simulink model "MicroMouseTemplate"  (R2023a)
settings: Solver=FixedStepAuto  StartTime=0.0  StopTime=50  RelTol=1e-3  EnableMultiTasking=on
undefined symbols (not defined in the file or in its folder): samplingTime
settings Model: SimulationMode=external  ExtModeTrigDuration=10  Creator=JesseJabezArendse  LastModifiedBy=Dylan Howard
settings SolverCC: AllowMultiTaskInputOutput=on  AutoInsertRateTranBlk=on  InsertRTBMode=Never (minimum delay)
settings OptimizationCC: EnhancedBackFolding=on  PassReuseOutputArgsAs=Individual arguments  StateBitsets=on  DataBitsets=on  ZeroExternalMemoryAtStartup=off  ZeroInternalMemoryAtStartup=off  NoFixptDivByZeroProtection=on  MaxStackSize=64  OptimizeBlockOrder=speed  DifferentSizesBufferReuse=on  EfficientTunableParamExpr=on
settings DebuggingCC: MultiTaskCondExecSysMsg=none  ParameterOverflowMsg=none  ParameterPrecisionLossMsg=none  ParameterTunabilityLossMsg=error
settings HardwareCC: ProdBitPerPointer=32  ProdBitPerSizeT=32  ProdBitPerPtrDiffT=32  ProdLargestAtomicInteger=Long  ProdLargestAtomicFloat=Double  ProdWordSize=32  ProdLongLongMode=on  ProdHWDeviceType=ARM Compatible->ARM Cortex  TargetBitPerPointer=64  TargetBitPerSizeT=64  TargetBitPerPtrDiffT=64  TargetLongLongMode=on  TargetIntDivRoundTo=Zero  TargetEndianess=LittleEndian  TargetWordSize=64  TargetHWDeviceType=MATLAB Host
settings ModelReferenceCC: EnableParallelModelReferenceBuilds=on  ParallelModelReferenceMATLABWorkerInit=Copy Base Workspace  SupportModelReferenceSimTargetCustomCode=on
settings SFSimCC: MATLABDynamicMemAlloc=off  SimHardwareAcceleration=native
settings RTWCC: Description=Embedded Coder  SystemTargetFile=ert.tlc  HardwareBoard=STM32L4xx Based  TLCOptions=-p0 -aInlineSetEventsForThisBaseRateFcn=TLC_FALSE -aSuppressMultiTaskScheduler=TLC_FALSE -aRateBasedStepFcn=1  TemplateMakefile=ert_default_tmf  Toolchain=GNU Tools for ARM Embedded Processors  CodeExecutionProfiling=on  CodeProfilingInstrumentation=coarse
settings RTWCC: CustomHeaderCode=|
  | #include "MicroMouseProgramming\Core\Inc\IMU.h"
  | #include "MicroMouseProgramming\Core\Inc\CustomWhile.h"
  | #include "MicroMouseProgramming\Core\Inc\Motors.h"
settings RTWCC: CustomInclude=|
  | MicroMouseProgramming\Core\Inc\
  | MicroMouseProgramming\Core\Src\
settings RTWCC: CustomSource=|
  | MicroMouseProgramming\Core\Src\IMU.c
  | MicroMouseProgramming\Core\Src\CustomWhile.c
  | MicroMouseProgramming\Core\Src\Motors.c
settings CodeAppCC: ForceParamTrailComments=on  IgnoreCustomStorageClasses=off  OperatorAnnotations=on  SimulinkDataObjDesc=on  SFDataObjDesc=on  InsertBlockDesc=on
settings ERTTargetCC: CodeReplacementLibrary=ARM Cortex-M  SupportNonFinite=off  SupportComplex=off  ExtModeTransport=3  ExtModeStaticAlloc=on  ExtModeStaticAllocSize=2048  ExtModeMexFile=ext_xcp  ExtModeIntrfLevel=Level2 - Open

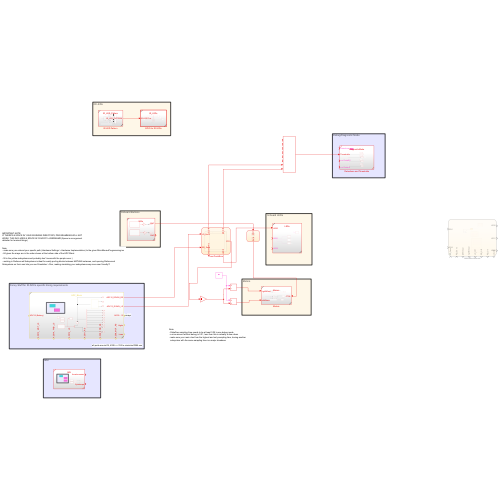
[thumbnail: Simulink's stored preview of the top-level diagram]
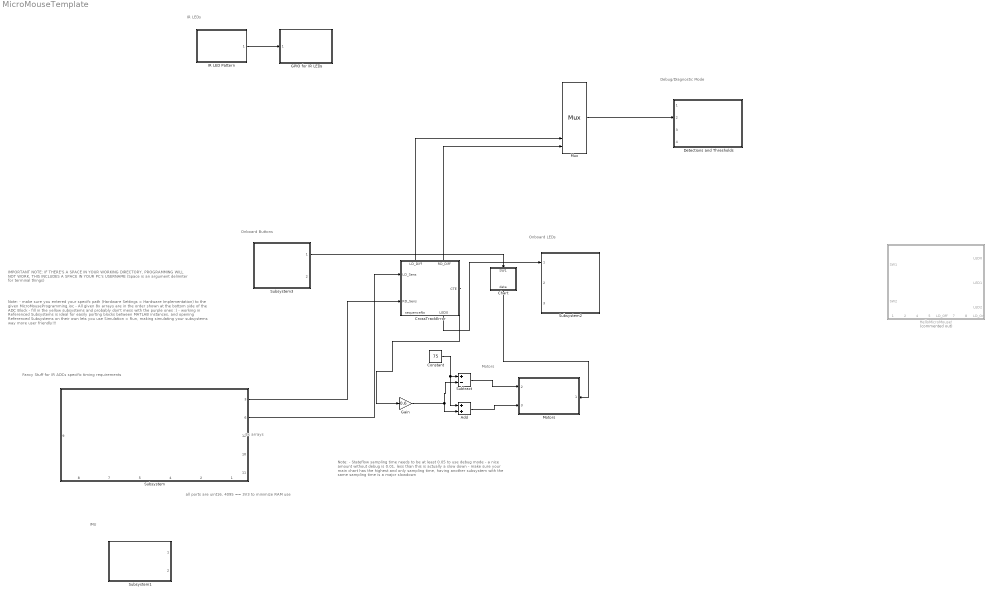
== system MicroMouseTemplate ==
  note: IMPORTANT NOTE:
      | IF THERE'S A SPACE IN YOUR WORKING DIRECTORY, PROGRAMMING WILL NOT WORK, THIS INCLUDES A SPACE IN YOUR PC's USERNAME (Space is an argument delimiter for terminal things)
  note: Note:
      | - make sure you entered your specifc path (Hardware Settings > Hardware Implementation) to the given MicroMouseProgramming.ioc
      | - All given 8x arrays are in the order shown at the bottom side of the ADC Block
      |
      | - fill in the yellow subsystems and probably don't mess with the purple ones :)
      | - working in Referenced Subsystems is ideal for easily porting blocks between MATLAB instances, and opening Referenced Subsystems on their own lets you use Simulation > Run, making simulating your subsystems way more user friendly!!!
  note: 8x arrays
  note: all ports are uint16, 4095 == 3V3 to minimize RAM use
  note: IMU
  note: Note:
      | - Stateflow sampling time needs to be at least 0.05 to use debug mode
      | - a nice amount without debug is 0.01, less than this is actually a slow down
      | - make sure your main chart has the highest and only sampling time, having another
      | subsystem with the same sampling time is a major slowdown
  note: Fancy Stuff for IR ADCs specific timing requirements
  note: IR LEDs
  note: Motors
  note: Onboard Buttons
  note: Onboard LEDs
  note: Debug/Diagnostic Mode
  Add : Sum
  Chart : Stateflow chart  TreatAsAtomicUnit=on
      settings: PortSchema="{\"entries\":[{\"content\":{\"sides\":[{\"content\":{},\"type\":\"ConnectorPlacement.EquallySpacedRectSide\",\"uuid\":\"65ce9c31-f788-4c01-8003-f22def2aa1a8\"},{\"content\":{\"side\":\"RIGHT\"},\"type\":\"ConnectorPlacement.EquallySpacedRectSide\",\"uuid\":\"9abbc0da-d05e-45e1-a3c7-84c2424ccecc\"},{\"content\":{\"connectorIds\":[\"In1\"],\"side\":\"TOP\"},\"type\":\"ConnectorPlacement.EquallySpacedRectSide\",\"uuid\":\"b07b8d41-8626-4028-b582-319b05f0b62f\"},{\"content\":{\"connectorIds\":[\"Out1\"],\"side\":\"BOTTOM\"},\"type\":\"ConnectorPlacement.EquallySpacedRectSide\",\"uuid\":\"589cd615-726f-470e-855b-ed4cc8a2624f\"}]},\"type\":\"ConnectorPlacement.EquallySpacedConnector\",\"uuid\":\"8c19fd69-3b5c-4f95-8b68-6f23bb3e3532\"}],\"packageUris\":[\"http://schema.mathworks.com/mf0/Connector/R2020b\"],\"version\":\"1.0\"}"
  Constant : Constant  Value=75
  CrossTrackError : Stateflow chart  TreatAsAtomicUnit=on
      settings: PortSchema="{\"entries\":[{\"content\":{\"sides\":[{\"content\":{\"connectorIds\":[\"In1\",\"In2\"]},\"type\":\"ConnectorPlacement.EquallySpacedRectSide\",\"uuid\":\"795ea1b7-921f-42f3-b63d-1e0fccd103e5\"},{\"content\":{\"connectorIds\":[\"Out1\"],\"side\":\"RIGHT\"},\"type\":\"ConnectorPlacement.EquallySpacedRectSide\",\"uuid\":\"448275bb-5ec0-437a-85f9-7eb442edc8cf\"},{\"content\":{\"connectorIds\":[\"Out5\",\"Out4\"],\"side\":\"TOP\"},\"type\":\"ConnectorPlacement.EquallySpacedRectSide\",\"uuid\":\"6cd8f479-822f-466b-98cd-321faa207bbc\"},{\"content\":{\"connectorIds\":[\"Out2\",\"Out3\"],\"side\":\"BOTTOM\"},\"type\":\"ConnectorPlacement.EquallySpacedRectSide\",\"uuid\":\"a7c78362-8d32-4585-892e-bb77329a6113\"}]},\"type\":\"ConnectorPlacement.EquallySpacedConnector\",\"uuid\":\"edaa4abf-4d20-4f3d-817e-a4fd7b08cb87\"}],\"packageUris\":[\"http://schema.mathworks.com/mf0/Connector/R2020b\"],\"version\":\"1.0\"}"
  Detections and Thresholds : Subsystem  ReferencedSubsystem=DiagnosticMode
  GPIO for IR LEDs : Subsystem  TreatAsAtomicUnit=on  SystemSampleTime=samplingTime  ReferencedSubsystem=IR_LEDs
  Gain : Gain  Gain=0.6
  HelloMicroMouse! : Stateflow chart  Commented=on  TreatAsAtomicUnit=on
      settings: PortSchema="{\"entries\":[{\"content\":{\"sides\":[{\"content\":{\"connectorIds\":[\"In4\",\"In3\"]},\"type\":\"ConnectorPlacement.EquallySpacedRectSide\",\"uuid\":\"f52daa4f-6374-42e5-9ef1-0ccc99d09b58\"},{\"content\":{\"connectorIds\":[\"Out1\",\"Out2\",\"Out3\"],\"side\":\"RIGHT\"},\"type\":\"ConnectorPlacement.EquallySpacedRectSide\",\"uuid\":\"94b478cc-4dde-45c7-a588-77cf2b43cdb7\"},{\"content\":{\"side\":\"TOP\"},\"type\":\"ConnectorPlacement.EquallySpacedRectSide\",\"uuid\":\"afff2079-ea5c-423e-9722-09c3bbce433b\"},{\"content\":{\"connectorIds\":[\"In1\",\"In2\",\"Out4\",\"Out5\",\"Out6\",\"Out7\",\"Out8\",\"Out9\"],\"side\":\"BOTTOM\"},\"type\":\"ConnectorPlacement.EquallySpacedRectSide\",\"uuid\":\"94e93a1d-795d-41a3-b2d8-d520b2bf47ef\"}]},\"type\":\"ConnectorPlacement.EquallySpacedConnector\",\"uuid\":\"d4d35636-54af-48ac-af70-d56caef5e090\"}],\"packageUris\":[\"http://schema.mathworks.com/mf0/Connector/R2020b\"],\"version\":\"1.0\"}"
  IR LED Pattern : Subsystem  ReferencedSubsystem=IR_LED_Pattern
  Motors : Subsystem  ReferencedSubsystem=Motors
      settings: PortSchema="{\"entries\":[{\"content\":{\"sides\":[{\"content\":{\"connectorIds\":[\"In2\",\"In3\"]},\"type\":\"ConnectorPlacement.EquallySpacedRectSide\",\"uuid\":\"524d3d59-9c7b-4144-8d0e-19eaf862ffe8\"},{\"content\":{\"connectorIds\":[\"In1\"],\"side\":\"RIGHT\"},\"type\":\"ConnectorPlacement.EquallySpacedRectSide\",\"uuid\":\"124526cf-9c70-4cc1-bf01-8ec9c9325922\"},{\"content\":{\"side\":\"TOP\"},\"type\":\"ConnectorPlacement.EquallySpacedRectSide\",\"uuid\":\"f46aa09a-ea93-4883-b41d-9c8b0d686de1\"}]},\"type\":\"ConnectorPlacement.EquallySpacedConnector\",\"uuid\":\"ff9f71c0-8007-42c1-ad0f-b0b809a6fe21\"}],\"packageUris\":[\"http://schema.mathworks.com/mf0/Connector/R2020b\"],\"version\":\"1.0\"}"
  Mux : Mux  Inputs=8
  Subsystem : Subsystem  ReferencedSubsystem=ADC_Block
      settings: PortSchema="{\"entries\":[{\"content\":{\"sides\":[{\"content\":{},\"type\":\"ConnectorPlacement.EquallySpacedRectSide\",\"uuid\":\"be6b81d5-7a49-4e34-b35f-0c07892094fc\"},{\"content\":{\"connectorIds\":[\"Out1\",\"Out2\",\"Out4\",\"Out5\",\"Out7\",\"Out8\"],\"side\":\"RIGHT\"},\"type\":\"ConnectorPlacement.EquallySpacedRectSide\",\"uuid\":\"5e22590a-b7c0-4c63-8de4-8d81fd6c3849\"},{\"content\":{\"connectorIds\":[\"Out3\",\"Out6\",\"Out12\",\"Out10\",\"Out11\"],\"side\":\"TOP\"},\"type\":\"ConnectorPlacement.EquallySpacedRectSide\",\"uuid\":\"da97636e-cea0-4a10-8fe5-d807f9ee999f\"},{\"content\":{\"connectorIds\":[\"Out9\"],\"side\":\"BOTTOM\"},\"type\":\"ConnectorPlacement.EquallySpacedRectSide\",\"uuid\":\"a593d780-81a8-4730-a8bc-2bbf356cafe4\"}]},\"type\":\"ConnectorPlacement.EquallySpacedConnector\",\"uuid\":\"0bcac921-e51a-4437-9183-315712d0a8c2\"}],\"packageUris\":[\"http://schema.mathworks.com/mf0/Connector/R2020b\"],\"version\":\"1.0\"}"
  Subsystem1 : Subsystem  ReferencedSubsystem=IMU
  Subsystem2 : Subsystem  ReferencedSubsystem=LEDs
  Subsystem3 : Subsystem  ReferencedSubsystem=SWs
  Subtract : Sum  Inputs=+-
  wires:
  Mux/1 -> Detections and Thresholds/2
  IR LED Pattern/1 -> GPIO for IR LEDs/1
  CrossTrackError/3(LED0) -> Subsystem2/1
  Subsystem/3 -> CrossTrackError/2(RD_Sens)
  Subsystem/6 -> CrossTrackError/1(LD_Sens)
  Chart/1(data) -> Motors/1
  Subsystem3/1 -> Chart/1(SW1)
  Subtract/1 -> Motors/2
  Constant/1 -> Add/1, Subtract/1
  Add/1 -> Motors/3
  CrossTrackError/1(CTE) -> Gain/1
  CrossTrackError/4(RD_Diff) -> Mux/8
  CrossTrackError/5(LD_Diff) -> Mux/7
  Gain/1 -> Subtract/2, Add/2

== stateflow chart MicroMouseTemplate/Chart ==
  state MotorCtrl
    entry:
  state MotorOn
    entry:
    data = 1;
  (default) -> MotorCtrl
  MotorCtrl -> MotorOn : [SW1]
  data: data output; SW1 input

== stateflow chart MicroMouseTemplate/HelloMicroMouse! ==
  state LEDPattern [commented out]
    entry:
    state Frame1 [commented out]
      entry:
      LED0 = 1;
      LED1 = 0;
      LED2= 0;
    state Frame2 [commented out]
      entry:
      LED0 = 0;
      LED1 = 1;
      LED2= 0;
    state Frame3 [commented out]
      entry:
      LED0 = 0;
      LED1 = 0;
      LED2= 1;
    (default) -> Frame1 [commented out]
    Frame1 -> Frame2 [commented out] : [after(0.3, sec)]
    Frame2 -> Frame3 [commented out] : [after(0.3, sec)]
    Frame3 -> Frame1 [commented out] : [after(0.3, sec)]
  state WaitTillButtonPress
    entry:
    LED0 = 0;
    LED1 = 0;
    LED2 = 0;
    leftWheel = 0;
    rightWheel = 0;
  state Calibrate [commented out]
    entry:
    LD_Max = 0;
    LD_Min = 4095;
    RD_Max = 0;
    RD_Min = 4095;
    state FindLimits [commented out]
      entry, during:
      if LD_Sens < LD_Min
      LD_Min = LD_Sens;
      end
      if LD_Sens > LD_Max
      LD_Max = LD_Sens;
      end
      if RD_Sens < RD_Min
      RD_Min = RD_Sens;
      end
      if RD_Sens > RD_Max
      RD_Max = RD_Sens;
      end
    state Blink [commented out]
      entry:
      if LED0
      LED0 = 0;
      else
      LED0 = 1;
      end
    (default) -> FindLimits [commented out]
    FindLimits -> Blink [commented out] : [after(0.5, sec)]
    Blink -> FindLimits [commented out]
  state WriteToDebug [commented out]
    entry:
    state WaitTillButtonPress [commented out]
      entry, during:
      LD_Norm =  uint16(4095*double(LD_Sens - LD_Min)/double(LD_Max - LD_Min));
      RD_Norm = uint16(4095*double(RD_Sens - RD_Min)/double(RD_Max - RD_Min));
      if LD_Norm <2500
      LED0 = 1;
      else
      LED0 = 0;
      end
      if RD_Norm < 4000
      LED2 = 1;
      else
      LED2 = 0;
      end
      if (RD_Norm < 4000)&&(LD_Norm < 2500)
      LED1 = 1;
      else
      LED1 = 0;
      end
    state WRite [commented out]
      entry, during:
      LD_Norm =  uint16(4095*double(LD_Sens - LD_Min)/double(LD_Max - LD_Min));
      RD_Norm = uint16(4095*double(RD_Sens - RD_Min)/double(RD_Max - RD_Min));
      if LD_Norm < 2500
      LED0 = 1;
      rightWheel = 75;
      leftWheel = 0;
      else
      LED0 = 0;
      end
      if RD_Norm < 4000
      LED2 = 1;
      rightWheel = 0;
      leftWheel = 75;
      else
      LED2 = 0;
      end
      if (RD_Norm < 4000)&&(LD_Norm < 2500)
      rightWheel = 75;
      leftWheel = 75;
      LED1 = 1;
      else
      LED1 = 0;
      end
    (default) -> WriteToDebug.WaitTillButtonPress [commented out]
    WriteToDebug.WaitTillButtonPress -> WRite [commented out] : [SW2]
  WaitTillButtonPress -> LEDPattern [commented out] : [SW1]
  (default) -> WaitTillButtonPress
  WaitTillButtonPress -> (junction 89) : [SW1]
  (junction 89) -> (junction 90)
  WaitTillButtonPress -> Calibrate [commented out] : [SW1]
  (junction 90) -> (junction 92) [order 1] : [after(2*0.2/3, sec)]
  (junction 90) -> (junction 94) [order 2]
  (junction 92) -> (junction 110) : {LD_On = LD_Sens;}
  (junction 94) -> (junction 96) [order 1] : [after(0.2/3, sec)]
  (junction 94) -> (junction 98) [order 2] : {LD_Off = LD_Sens;
      | RD_Off = RD_Sens;}
  (junction 96) -> (junction 112) : {RD_On = RD_Sens;}
  (junction 112) -> (junction 98)
  (junction 110) -> (junction 112)
  Calibrate -> WriteToDebug [commented out] : [after(30, sec)]
  data: LD_Sens input; RD_Sens input; SW2 input; LED0 output; LED1 output; LED2 output; SW1 input; leftWheel output int8; rightWheel output int8; RD_Min local uint16; RD_Max local uint16; LD_Min local uint16; LD_Max local uint16; LD_Off output; RD_Off output; RD_On output; LD_On output

== stateflow chart MicroMouseTemplate/CrossTrackError ==
  state One
    entry:
    RD_Diff = 175;
    LD_Diff = 175;
    sequenceNo = 2;
    LD_On = 0;
    RD_On = 0;
    LD_Off = 0;
    RD_Off = 0;
    LED0 = 0;
    CTE = 0;
    CrossOverCount = 0;
    state getVals
      during:
      sequenceNo = sequenceNo + 1;
      if sequenceNo == 3
      sequenceNo = 0;
      end
      if sequenceNo == 0
      LD_Off = LD_Sens;
      RD_Off = RD_Sens;
      end
      if sequenceNo == 1
      LD_On = LD_Sens;
      end
      if sequenceNo == 2
      RD_On = RD_Sens;
      RD_Diff   =  max(min(1.5*((RD_On  -  RD_Off)), 175), 75);
      LD_Diff    =  max(min(9*(LD_On  -  LD_Off), 175), 75);
      CTE = double(RD_Diff) - double(LD_Diff);
      end
      if (LD_Diff < 80) && (RD_Diff < 80)
      CrossOverCount =  CrossOverCount + 1;
      if(CrossOverCount > 20)
      if LED0 == 1
      LED0 = 0;
      else
      LED0 = 1;
      end
      CrossOverCount = 0;
      end
      end
    (default) -> getVals
  (default) -> One
  data: CTE output double; sequenceNo output uint16; LD_Sens input; LED0 output; RD_Sens input; LD_Sum local; RD_Sum local; RD_On local uint16; RD_Off local uint16; LD_On local uint16; LD_Off local uint16; RD_Diff output uint16; LD_Diff output uint16; CrossOverCount local
